simulink model "volo_radio_controller"  (Simulink 8.0)
settings: Solver=ode45  SolverMode=SingleTasking  StartTime=0.0  StopTime=1000  RelTol=1e-3
InitFcn:
  | volo_radio_controller_init
values from neighbouring files (symbols this model uses):
  cFI = fi(cMult, 1, 13, 11)    [volo_radio_controller_init.m]
  gFI = fi(gain, 1, 13, 11)    [volo_radio_controller_init.m]
  sFI = fi(sMult, 1, 13, 11)    [volo_radio_controller_init.m]
undefined symbols (not defined in the file or in its folder): gcbh, xlBlockLoadCallback, xlGetNormalizedPeriod, xlipgetpartsetting
libraries: xbsIndex_r4 x380, xbsEDKLib_r4 x1
(part 5 of 5)

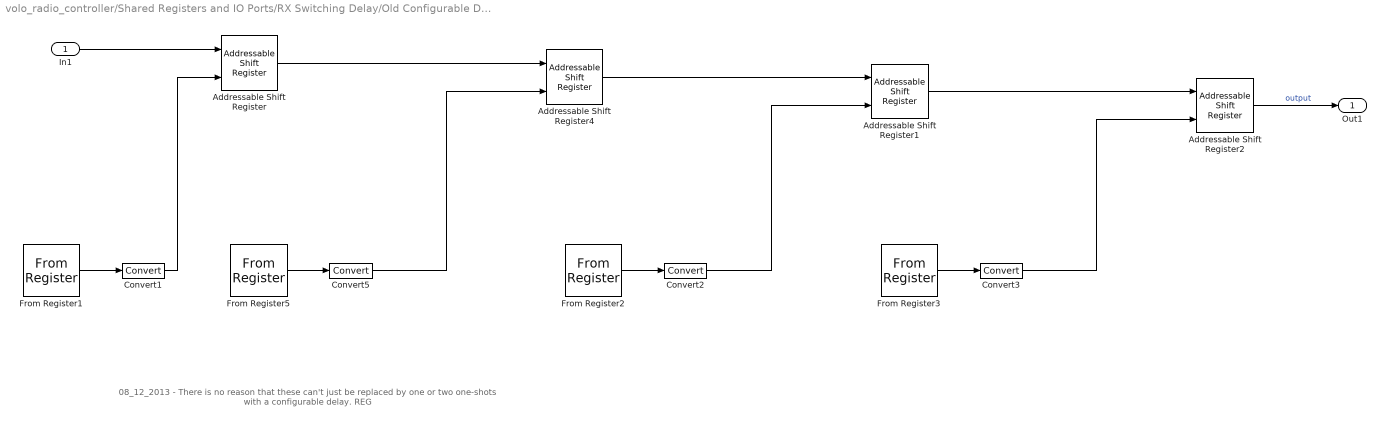
== system volo_radio_controller/Shared Registers and IO Ports/RX Switching Delay/Old Configurable Delay Block ==
  note: 08_12_2013 - There is no reason that these can't just be replaced by one or two one-shots with a configurable delay. REG
  In1 : Inport
  Addressable Shift Register{,1..2,4} (4 alike) : xbsIndex_r4/Addressable Shift Register  infer_latency=off  depth=1024  initVector=[0]  en=off  dbl_ovrd=off  use_behavioral_HDL=off  Optimization=Resource  block_type=addrsr
      settings: infoedit="Delay of configurable length.  Any element in the delay line can be addressed and driven onto the output port.<br><br>Hardware notes: This block is implemented using SRL16s. If Virtex-4 or Spartan-3 device is used, multiple SRLC16s are cascaded together."
  Convert{1..3,5} (4 alike) : xbsIndex_r4/Convert  gui_display_data_type=Fixed-point  arith_type=Unsigned  n_bits=10  bin_pt=0  float_type=Single  exp_bits=8  fraction_bits=24  quantization=Truncate  overflow=Saturate  en=off  latency=0  dbl_ovrd=off  pipeline=off  block_type=convert
  From Register1 : xbsIndex_r4/From Register  shared_memory_name='VOLO_TX_EN_DLY'  init=0  period=1  ownership=Locally owned and initialized  gui_display_data_type=Fixed-point  arith_type=Unsigned  n_bits=32  bin_pt=0  preci_type=Single  dbl_ovrd=off  block_type=fromreg
      settings: AttributesFormatString=<< %<shared_memory_name> >>  infoedit="Register block that reads data to a shared memory register.  Delay of one sample period."
  From Register2 : xbsIndex_r4/From Register  shared_memory_name='VOLO_TX_EN_DLY3'  init=0  period=1  ownership=Locally owned and initialized  gui_display_data_type=Fixed-point  arith_type=Unsigned  n_bits=32  bin_pt=0  preci_type=Single  dbl_ovrd=off  block_type=fromreg
      settings: AttributesFormatString=<< %<shared_memory_name> >>  infoedit="Register block that reads data to a shared memory register.  Delay of one sample period."
  From Register3 : xbsIndex_r4/From Register  shared_memory_name='VOLO_TX_EN_DLY4'  init=0  period=1  ownership=Locally owned and initialized  gui_display_data_type=Fixed-point  arith_type=Unsigned  n_bits=32  bin_pt=0  preci_type=Single  dbl_ovrd=off  block_type=fromreg
      settings: AttributesFormatString=<< %<shared_memory_name> >>  infoedit="Register block that reads data to a shared memory register.  Delay of one sample period."
  From Register5 : xbsIndex_r4/From Register  shared_memory_name='VOLO_TX_EN_DLY2'  init=0  period=1  ownership=Locally owned and initialized  gui_display_data_type=Fixed-point  arith_type=Unsigned  n_bits=32  bin_pt=0  preci_type=Single  dbl_ovrd=off  block_type=fromreg
      settings: AttributesFormatString=<< %<shared_memory_name> >>  infoedit="Register block that reads data to a shared memory register.  Delay of one sample period."
  Out1 : Outport
  wires:
  Addressable Shift Register4/1 -> Addressable Shift Register1/1
  Addressable Shift Register2/1 -> Out1/1  "output"
  From Register2/1 -> Convert2/1
  From Register3/1 -> Convert3/1
  Convert2/1 -> Addressable Shift Register1/2
  Convert3/1 -> Addressable Shift Register2/2
  Convert5/1 -> Addressable Shift Register4/2
  From Register1/1 -> Convert1/1
  Addressable Shift Register/1 -> Addressable Shift Register4/1
  Convert1/1 -> Addressable Shift Register/2
  Addressable Shift Register1/1 -> Addressable Shift Register2/1
  From Register5/1 -> Convert5/1
  In1/1 -> Addressable Shift Register/1

== system volo_radio_controller/Shared Registers and IO Ports/RX Switching Delay/rising edge ==
  note: rising edge
  A : Inport
  Delay1 : xbsIndex_r4/Delay  rst=off  infoeditControl=Selection of Reset will increase slice count due to use of real FFs and instead of SRLs  en=off  latency=1  dbl_ovrd=off  reg_retiming=off  block_type=delay
  Inverter2 : xbsIndex_r4/Inverter  en=off  latency=0  dbl_ovrd=off  block_type=inv
  Logical2 : xbsIndex_r4/Logical  logical_function=AND  inputs=2  en=off  latency=0  precision=Full  arith_type=Unsigned  n_bits=16  bin_pt=0  align_bp=on  dbl_ovrd=off  block_type=logical
  Q : Outport
  wires:
  Logical2/1 -> Q/1
  A/1 -> Logical2/1, Delay1/1
  Delay1/1 -> Inverter2/1
  Inverter2/1 -> Logical2/2

== system volo_radio_controller/Shared Registers and IO Ports/SPI Flush Delay /32Bit_OneShot ==
  Start : Inport
  CountTo : Inport  Port=2
  RST : Inport  Port=3
  HoldUntilReset : Subsystem
  Inverter2 : xbsIndex_r4/Inverter  en=off  latency=0  dbl_ovrd=off  block_type=inv
  Logical5 : xbsIndex_r4/Logical  logical_function=AND  inputs=2  en=off  latency=0  precision=Full  arith_type=Unsigned  n_bits=16  bin_pt=0  align_bp=on  dbl_ovrd=off  block_type=logical
  PayloadTimeoutCounter : xbsIndex_r4/Counter  cnt_type=Free Running  cnt_to=Inf  operation=Up  start_count=0  cnt_by_val=1  arith_type=Unsigned  n_bits=32  bin_pt=0  load_pin=off  rst=on  en=on  explicit_period=on  period=1  dbl_ovrd=off  use_behavioral_HDL=off  implementation=Fabric  block_type=counter
  Relational2 : xbsIndex_r4/Relational  mode=a=b  en=off  latency=0  dbl_ovrd=off  block_type=relational
  Done : Outport
  wires:
  RST/1 -> HoldUntilReset/2(RST), PayloadTimeoutCounter/1
  CountTo/1 -> Relational2/2
  PayloadTimeoutCounter/1 -> Relational2/1
  Relational2/1 -> Inverter2/1, Done/1  "payloadTimeout"
  Inverter2/1 -> Logical5/2
  Logical5/1 -> PayloadTimeoutCounter/2
  Start/1 -> HoldUntilReset/1(A)
  HoldUntilReset/1(Q) -> Logical5/1

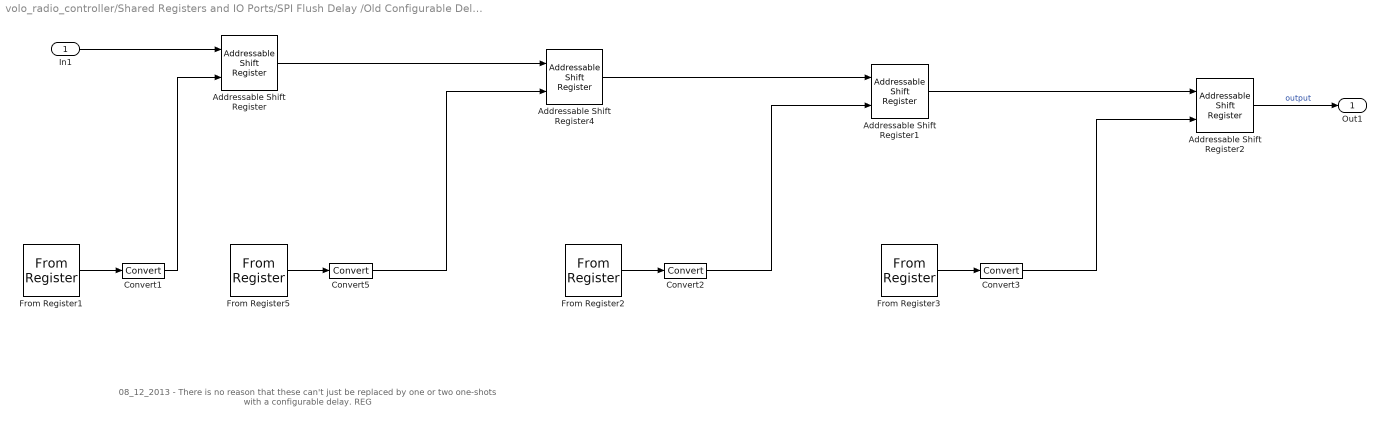
== system volo_radio_controller/Shared Registers and IO Ports/SPI Flush Delay /Old Configurable Delay Block ==
  note: 08_12_2013 - There is no reason that these can't just be replaced by one or two one-shots with a configurable delay. REG
  In1 : Inport
  Addressable Shift Register{,1..2,4} (4 alike) : xbsIndex_r4/Addressable Shift Register  infer_latency=off  depth=1024  initVector=[0]  en=off  dbl_ovrd=off  use_behavioral_HDL=off  Optimization=Resource  block_type=addrsr
      settings: infoedit="Delay of configurable length.  Any element in the delay line can be addressed and driven onto the output port.<br><br>Hardware notes: This block is implemented using SRL16s. If Virtex-4 or Spartan-3 device is used, multiple SRLC16s are cascaded together."
  Convert{1..3,5} (4 alike) : xbsIndex_r4/Convert  gui_display_data_type=Fixed-point  arith_type=Unsigned  n_bits=10  bin_pt=0  float_type=Single  exp_bits=8  fraction_bits=24  quantization=Truncate  overflow=Saturate  en=off  latency=0  dbl_ovrd=off  pipeline=off  block_type=convert
  From Register1 : xbsIndex_r4/From Register  shared_memory_name='VOLO_TX_EN_DLY'  init=0  period=1  ownership=Locally owned and initialized  gui_display_data_type=Fixed-point  arith_type=Unsigned  n_bits=32  bin_pt=0  preci_type=Single  dbl_ovrd=off  block_type=fromreg
      settings: AttributesFormatString=<< %<shared_memory_name> >>  infoedit="Register block that reads data to a shared memory register.  Delay of one sample period."
  From Register2 : xbsIndex_r4/From Register  shared_memory_name='VOLO_TX_EN_DLY3'  init=0  period=1  ownership=Locally owned and initialized  gui_display_data_type=Fixed-point  arith_type=Unsigned  n_bits=32  bin_pt=0  preci_type=Single  dbl_ovrd=off  block_type=fromreg
      settings: AttributesFormatString=<< %<shared_memory_name> >>  infoedit="Register block that reads data to a shared memory register.  Delay of one sample period."
  From Register3 : xbsIndex_r4/From Register  shared_memory_name='VOLO_TX_EN_DLY4'  init=0  period=1  ownership=Locally owned and initialized  gui_display_data_type=Fixed-point  arith_type=Unsigned  n_bits=32  bin_pt=0  preci_type=Single  dbl_ovrd=off  block_type=fromreg
      settings: AttributesFormatString=<< %<shared_memory_name> >>  infoedit="Register block that reads data to a shared memory register.  Delay of one sample period."
  From Register5 : xbsIndex_r4/From Register  shared_memory_name='VOLO_TX_EN_DLY2'  init=0  period=1  ownership=Locally owned and initialized  gui_display_data_type=Fixed-point  arith_type=Unsigned  n_bits=32  bin_pt=0  preci_type=Single  dbl_ovrd=off  block_type=fromreg
      settings: AttributesFormatString=<< %<shared_memory_name> >>  infoedit="Register block that reads data to a shared memory register.  Delay of one sample period."
  Out1 : Outport
  wires:
  Addressable Shift Register4/1 -> Addressable Shift Register1/1
  Addressable Shift Register2/1 -> Out1/1  "output"
  From Register2/1 -> Convert2/1
  From Register3/1 -> Convert3/1
  Convert2/1 -> Addressable Shift Register1/2
  Convert3/1 -> Addressable Shift Register2/2
  Convert5/1 -> Addressable Shift Register4/2
  From Register1/1 -> Convert1/1
  Addressable Shift Register/1 -> Addressable Shift Register4/1
  Convert1/1 -> Addressable Shift Register/2
  Addressable Shift Register1/1 -> Addressable Shift Register2/1
  From Register5/1 -> Convert5/1
  In1/1 -> Addressable Shift Register/1

== system volo_radio_controller/Shared Registers and IO Ports/SPI Flush Delay /rising edge ==
  note: rising edge
  A : Inport
  Delay1 : xbsIndex_r4/Delay  rst=off  infoeditControl=Selection of Reset will increase slice count due to use of real FFs and instead of SRLs  en=off  latency=1  dbl_ovrd=off  reg_retiming=off  block_type=delay
  Inverter2 : xbsIndex_r4/Inverter  en=off  latency=0  dbl_ovrd=off  block_type=inv
  Logical2 : xbsIndex_r4/Logical  logical_function=AND  inputs=2  en=off  latency=0  precision=Full  arith_type=Unsigned  n_bits=16  bin_pt=0  align_bp=on  dbl_ovrd=off  block_type=logical
  Q : Outport
  wires:
  Logical2/1 -> Q/1
  A/1 -> Logical2/1, Delay1/1
  Delay1/1 -> Inverter2/1
  Inverter2/1 -> Logical2/2

== system volo_radio_controller/Shared Registers and IO Ports/TX Switching Delay/32Bit_OneShot ==
  Start : Inport
  CountTo : Inport  Port=2
  RST : Inport  Port=3
  HoldUntilReset : Subsystem
  Inverter2 : xbsIndex_r4/Inverter  en=off  latency=0  dbl_ovrd=off  block_type=inv
  Logical5 : xbsIndex_r4/Logical  logical_function=AND  inputs=2  en=off  latency=0  precision=Full  arith_type=Unsigned  n_bits=16  bin_pt=0  align_bp=on  dbl_ovrd=off  block_type=logical
  PayloadTimeoutCounter : xbsIndex_r4/Counter  cnt_type=Free Running  cnt_to=Inf  operation=Up  start_count=0  cnt_by_val=1  arith_type=Unsigned  n_bits=32  bin_pt=0  load_pin=off  rst=on  en=on  explicit_period=on  period=1  dbl_ovrd=off  use_behavioral_HDL=off  implementation=Fabric  block_type=counter
  Relational2 : xbsIndex_r4/Relational  mode=a=b  en=off  latency=0  dbl_ovrd=off  block_type=relational
  Done : Outport
  wires:
  RST/1 -> HoldUntilReset/2(RST), PayloadTimeoutCounter/1
  CountTo/1 -> Relational2/2
  PayloadTimeoutCounter/1 -> Relational2/1
  Relational2/1 -> Inverter2/1, Done/1  "payloadTimeout"
  Inverter2/1 -> Logical5/2
  Logical5/1 -> PayloadTimeoutCounter/2
  Start/1 -> HoldUntilReset/1(A)
  HoldUntilReset/1(Q) -> Logical5/1

== system volo_radio_controller/Shared Registers and IO Ports/TX Switching Delay/Old Configurable Delay Block ==
  note: 08_12_2013 - There is no reason that these can't just be replaced by one or two one-shots with a configurable delay. REG
  In1 : Inport
  Addressable Shift Register{,1..2,4} (4 alike) : xbsIndex_r4/Addressable Shift Register  infer_latency=off  depth=1024  initVector=[0]  en=off  dbl_ovrd=off  use_behavioral_HDL=off  Optimization=Resource  block_type=addrsr
      settings: infoedit="Delay of configurable length.  Any element in the delay line can be addressed and driven onto the output port.<br><br>Hardware notes: This block is implemented using SRL16s. If Virtex-4 or Spartan-3 device is used, multiple SRLC16s are cascaded together."
  Convert{1..3,5} (4 alike) : xbsIndex_r4/Convert  gui_display_data_type=Fixed-point  arith_type=Unsigned  n_bits=10  bin_pt=0  float_type=Single  exp_bits=8  fraction_bits=24  quantization=Truncate  overflow=Saturate  en=off  latency=0  dbl_ovrd=off  pipeline=off  block_type=convert
  From Register1 : xbsIndex_r4/From Register  shared_memory_name='VOLO_TX_EN_DLY'  init=0  period=1  ownership=Locally owned and initialized  gui_display_data_type=Fixed-point  arith_type=Unsigned  n_bits=32  bin_pt=0  preci_type=Single  dbl_ovrd=off  block_type=fromreg
      settings: AttributesFormatString=<< %<shared_memory_name> >>  infoedit="Register block that reads data to a shared memory register.  Delay of one sample period."
  From Register2 : xbsIndex_r4/From Register  shared_memory_name='VOLO_TX_EN_DLY3'  init=0  period=1  ownership=Locally owned and initialized  gui_display_data_type=Fixed-point  arith_type=Unsigned  n_bits=32  bin_pt=0  preci_type=Single  dbl_ovrd=off  block_type=fromreg
      settings: AttributesFormatString=<< %<shared_memory_name> >>  infoedit="Register block that reads data to a shared memory register.  Delay of one sample period."
  From Register3 : xbsIndex_r4/From Register  shared_memory_name='VOLO_TX_EN_DLY4'  init=0  period=1  ownership=Locally owned and initialized  gui_display_data_type=Fixed-point  arith_type=Unsigned  n_bits=32  bin_pt=0  preci_type=Single  dbl_ovrd=off  block_type=fromreg
      settings: AttributesFormatString=<< %<shared_memory_name> >>  infoedit="Register block that reads data to a shared memory register.  Delay of one sample period."
  From Register5 : xbsIndex_r4/From Register  shared_memory_name='VOLO_TX_EN_DLY2'  init=0  period=1  ownership=Locally owned and initialized  gui_display_data_type=Fixed-point  arith_type=Unsigned  n_bits=32  bin_pt=0  preci_type=Single  dbl_ovrd=off  block_type=fromreg
      settings: AttributesFormatString=<< %<shared_memory_name> >>  infoedit="Register block that reads data to a shared memory register.  Delay of one sample period."
  Out1 : Outport
  wires:
  Addressable Shift Register4/1 -> Addressable Shift Register1/1
  Addressable Shift Register2/1 -> Out1/1  "output"
  From Register2/1 -> Convert2/1
  From Register3/1 -> Convert3/1
  Convert2/1 -> Addressable Shift Register1/2
  Convert3/1 -> Addressable Shift Register2/2
  Convert5/1 -> Addressable Shift Register4/2
  From Register1/1 -> Convert1/1
  Addressable Shift Register/1 -> Addressable Shift Register4/1
  Convert1/1 -> Addressable Shift Register/2
  Addressable Shift Register1/1 -> Addressable Shift Register2/1
  From Register5/1 -> Convert5/1
  In1/1 -> Addressable Shift Register/1

== system volo_radio_controller/Shared Registers and IO Ports/TX Switching Delay/rising edge ==
  note: rising edge
  A : Inport
  Delay1 : xbsIndex_r4/Delay  rst=off  infoeditControl=Selection of Reset will increase slice count due to use of real FFs and instead of SRLs  en=off  latency=1  dbl_ovrd=off  reg_retiming=off  block_type=delay
  Inverter2 : xbsIndex_r4/Inverter  en=off  latency=0  dbl_ovrd=off  block_type=inv
  Logical2 : xbsIndex_r4/Logical  logical_function=AND  inputs=2  en=off  latency=0  precision=Full  arith_type=Unsigned  n_bits=16  bin_pt=0  align_bp=on  dbl_ovrd=off  block_type=logical
  Q : Outport
  wires:
  Logical2/1 -> Q/1
  A/1 -> Logical2/1, Delay1/1
  Delay1/1 -> Inverter2/1
  Inverter2/1 -> Logical2/2

== system volo_radio_controller/Shared Registers and IO Ports/RX Switching Delay/32Bit_OneShot/HoldUntilReset ==
  A : Inport
  RST : Inport  Port=2
  Register : xbsIndex_r4/Register  init=0  rst=on  en=on  dbl_ovrd=off  block_type=register
  Q : Outport
  wires:
  RST/1 -> Register/2
  Register/1 -> Q/1
  A/1 -> Register/1, Register/3

== system volo_radio_controller/Shared Registers and IO Ports/SPI Flush Delay /32Bit_OneShot/HoldUntilReset ==
  A : Inport
  RST : Inport  Port=2
  Register : xbsIndex_r4/Register  init=0  rst=on  en=on  dbl_ovrd=off  block_type=register
  Q : Outport
  wires:
  RST/1 -> Register/2
  Register/1 -> Q/1
  A/1 -> Register/1, Register/3

== system volo_radio_controller/Shared Registers and IO Ports/TX Switching Delay/32Bit_OneShot/HoldUntilReset ==
  A : Inport
  RST : Inport  Port=2
  Register : xbsIndex_r4/Register  init=0  rst=on  en=on  dbl_ovrd=off  block_type=register
  Q : Outport
  wires:
  RST/1 -> Register/2
  Register/1 -> Q/1
  A/1 -> Register/1, Register/3
